simulink model "ss_model_compare_tf_model"  (R2015a)
settings: Solver=ode3  StartTime=0.0  StopTime=100  FixedStep=0.001  RelTol=1e-3
values from neighbouring files (symbols this model uses):
  b = 50    [cruise_control_ss.m]
undefined symbols (not defined in the file or in its folder): a, c, d
libraries: simulink_extras x1
settings Model: Creator=Xiaotian  LastModifiedBy=Xiaotian

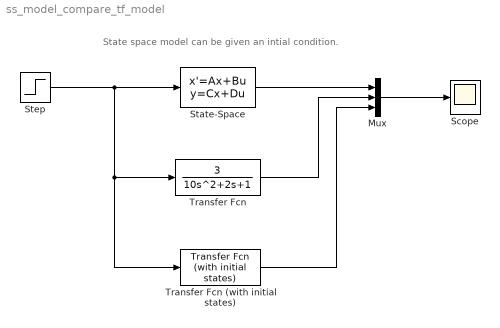
== system ss_model_compare_tf_model ==
  note: State space model can be given an intial condition.
  Mux : Mux  Inputs=3
  Scope : Scope
      settings: TimeRange=10  YMin=-3  YMax=6  SampleInput=on
  State-Space : StateSpace  A=a  B=b  C=c  D=d  X0=[0 1]
  Step : Step  Time=10  SampleTime=0
  Transfer Fcn : TransferFcn  Numerator=[3]  Denominator=[10 2 1]
  Transfer Fcn (with initial states) : simulink_extras/Additional Linear/Transfer Fcn (with initial states)  N=[3]  D=[10 2 1]  X0=[0.5]
  wires:
  Step/1 -> Transfer Fcn (with initial states)/1, Transfer Fcn/1, State-Space/1
  Mux/1 -> Scope/1
  State-Space/1 -> Mux/1
  Transfer Fcn/1 -> Mux/2
  Transfer Fcn (with initial states)/1 -> Mux/3
